simulink model "testinput2"  (Simulink 3.00)
settings: Solver=FixedStepDiscrete  StartTime=0.0  StopTime=60.0  FixedStep=0.02  RelTol=1e-3
settings Model: LastModifiedBy=hkg

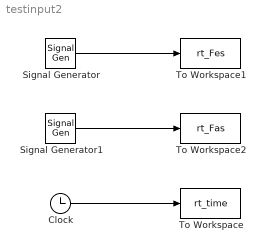
== system testinput2 ==
  Clock : Clock
      settings: DisplayTime=off  Decimation=10
  Signal Generator : SignalGenerator  WaveForm=sine  Amplitude=40  Frequency=0.2  Units=Hertz
  Signal Generator1 : SignalGenerator  WaveForm=sine  Amplitude=5  Frequency=0.3  Units=Hertz
  To Workspace : ToWorkspace  VariableName=rt_time  SampleTime=-1  SaveFormat=Matrix
  To Workspace1 : ToWorkspace  VariableName=rt_Fes  SampleTime=-1  SaveFormat=Matrix
  To Workspace2 : ToWorkspace  VariableName=rt_Fas  SampleTime=-1  SaveFormat=Matrix
  wires:
  Clock/1 -> To Workspace/1
  Signal Generator/1 -> To Workspace1/1
  Signal Generator1/1 -> To Workspace2/1
